simulink model "mpc_final"  (R2024a)
settings: Solver=ode4  StartTime=0  StopTime=5  FixedStep=0.25e-6  RelTol=1e-3
values from neighbouring files (symbols this model uses):
  B = 0    [PMSM_parameters.m]
  J = 0.006    [PMSM_parameters.m]
  Ls = 0.4    [PMSM_parameters.m]
  p = 4    [PMSM_parameters.m]
  Rs = 0.02    [PMSM_parameters.m]
  Sm = 0.2205    [PMSM_parameters.m]
libraries: slpidlib x4, embmathops x2, spsTHDLib x1
settings Model: NumberOfSteps=10  Creator=rohit  LastModifiedBy=rohit

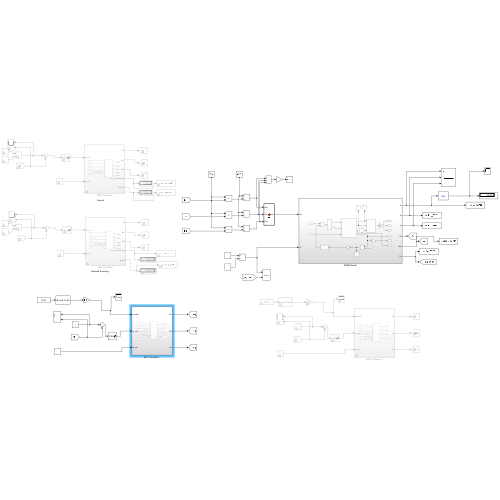
[thumbnail: Simulink's stored preview of the top-level diagram]
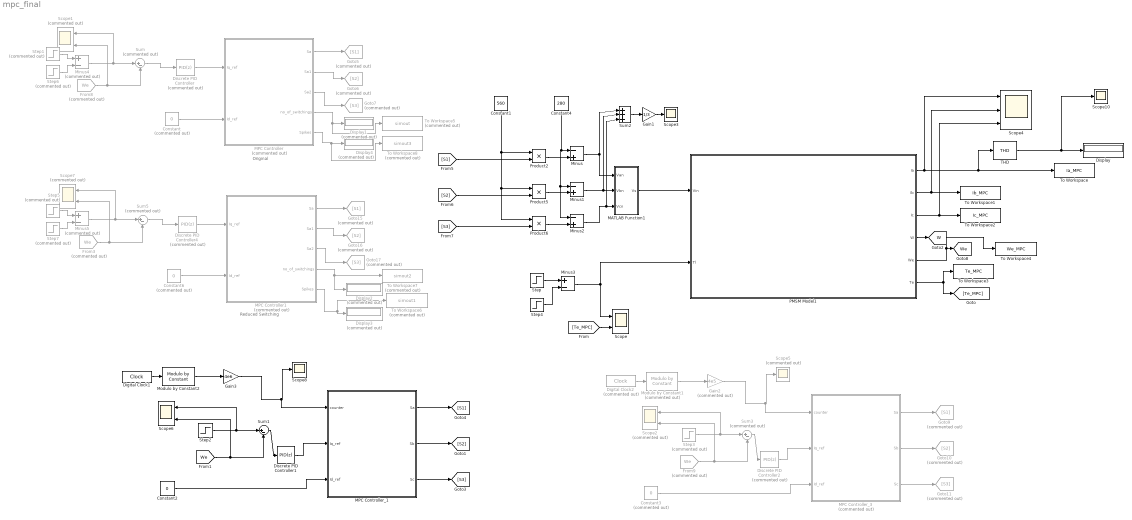
== system mpc_final ==
  note: Original
  note: Reduced Switching
  Constant : Constant  Commented=on  Value=0
  Constant1 : Constant  Value=560
  Constant2 : Constant  Value=0
  Constant3 : Constant  Commented=on  Value=0
  Constant4 : Constant  Value=280
  Constant6 : Constant  Commented=on  Value=0
  Digital Clock1 : DigitalClock  SampleTime=2.5e-6
  Digital Clock2 : DigitalClock  Commented=on  SampleTime=2.5e-6
  Discrete PID Controller : slpidlib/PID Controller  Commented=on  Controller=PID  Form=Parallel  TimeDomain=Discrete-time  UseExternalTs=off  SampleTime=-1  IntegratorMethod=Forward Euler  FilterMethod=Forward Euler  ControllerParametersSource=internal  P=10  I=1  UseKiTs=off  D=1  UseExternalDerivativeSource=off  N=100  UseFilter=off  TunerSelectOption=Transfer Function Based (PID Tuner App)  InitialConditionSource=internal  InitialConditionForIntegrator=0  InitialConditionForFilter=0  DifferentiatorICPrevScaledInput=0  ExternalReset=none  TrackingMode=off  Kt=1  LimitOutput=on  SatLimitsSource=internal  UpperSaturationLimit=90  LowerSaturationLimit=-90  LinearizeAsGain=on  AntiWindupMode=clamping  Kb=1  LimitIntegrator=off  UpperIntegratorSaturationLimit=inf  LowerIntegratorSaturationLimit=-inf  POutMin=[]  POutMax=[]  IOutMin=[]  IOutMax=[]  DOutMin=[]  DOutMax=[]  NOutMin=[]  NOutMax=[]  SumOutMin=[]  SumOutMax=[]  SaturationOutMin=[]  SaturationOutMax=[]  PParamMin=[]  PParamMax=[]  IParamMin=[]  IParamMax=[]  DParamMin=[]  DParamMax=[]  NParamMin=[]  NParamMax=[]  KbParamMin=[]  KbParamMax=[]  KtParamMin=[]  KtParamMax=[]  KbOutMin=[]  KbOutMax=[]  KtOutMin=[]  KtOutMax=[]  IntegratorOutMin=[]  IntegratorOutMax=[]  FilterOutMin=[]  FilterOutMax=[]  SumI1OutMin=[]  SumI1OutMax=[]  SumI2OutMin=[]  SumI2OutMax=[]  SumI3OutMin=[]  SumI3OutMax=[]  SumI4OutMin=[]  SumI4OutMax=[]  SumDOutMin=[]  SumDOutMax=[]  DifferentiatorOutMin=[]  DifferentiatorOutMax=[]  FilterDiffOutCoefMin=[]  FilterDiffOutCoefMax=[]  ReciprocalOutMin=[]  ReciprocalOutMax=[]  SumDenOutMin=[]  SumDenOutMax=[]  SumNumOutMin=[]  SumNumOutMax=[]  DivideOutMin=[]  DivideOutMax=[]  UdiffTsProdOutMin=[]  UdiffTsProdOutMax=[]  NTsProdOutMin=[]  NTsProdOutMax=[]  UintegralTsProdOutMin=[]  UintegralTsProdOutMax=[]  UngainTsProdOutMin=[]  UngainTsProdOutMax=[]  ClampingZeroOutDataTypeStr=Inherit: Inherit via back propagation  ClampingZeroOutMin=[]  ClampingZeroOutMax=[]  FilterDenConstantOutDataTypeStr=Inherit: Inherit via back propagation  FilterDenConstantOutMin=[]  FilterDenConstantOutMax=[]  PCopyOutDataTypeStr=Inherit: Inherit via back propagation  PCopyOutMin=[]  PCopyOutMax=[]  NCopyOutDataTypeStr=Inherit: Inherit via back propagation  NCopyOutMin=[]  NCopyOutMax=[]  IntegratorContinuousStateAttributes=''  IntegratorStateMustResolveToSignalObject=off  IntegratorRTWStateStorageClass=Auto  FilterContinuousStateAttributes=''  FilterStateMustResolveToSignalObject=off  FilterRTWStateStorageClass=Auto  ParallelPVariant=InternalParameters  IdealPVariant=Disabled  IVariant=InternalParameters  DVariant=InternalParameters  IntegratorVariant=Discrete  SatVariant=Enabled  AWVariant=DiscClampingParallel  PCopyVariant=Disabled  TRVariant=Disabled  FdbkBlocksVariant=Forward  IdealPFdbkVariant=Disabled  SatFdbkVariant=Disabled  DerivativeFilterVariant=Differentiator  NVariant=Passthrough  NCopyVariant=Disabled_SignalSpec  FilterICVariant=InternalICsDifferentiator  IntegratorICVariant=InternalICs  ExternalResetVariant=Disabled  TRSumVariant=Passthrough  SumFdbkVariant=Disabled  SumVariant=Sum_PID  TsampFilterVariant=InternalTs  TsampNgainVariant=Passthrough  TsampIntegralVariant=Disabled_SignalSpec  ExternalSaturationOutDataTypeStr=Inherit: Same as second input  DerivativeSourceVariant=ErrorSignal
  Discrete PID Controller1 : slpidlib/PID Controller  Controller=PID  Form=Parallel  TimeDomain=Discrete-time  UseExternalTs=off  SampleTime=-1  IntegratorMethod=Forward Euler  FilterMethod=Forward Euler  ControllerParametersSource=internal  P=10  I=1  UseKiTs=off  D=1  UseExternalDerivativeSource=off  N=100  UseFilter=off  TunerSelectOption=Transfer Function Based (PID Tuner App)  InitialConditionSource=internal  InitialConditionForIntegrator=0  InitialConditionForFilter=0  DifferentiatorICPrevScaledInput=0  ExternalReset=none  TrackingMode=off  Kt=1  LimitOutput=on  SatLimitsSource=internal  UpperSaturationLimit=90  LowerSaturationLimit=-90  LinearizeAsGain=on  AntiWindupMode=clamping  Kb=1  LimitIntegrator=off  UpperIntegratorSaturationLimit=inf  LowerIntegratorSaturationLimit=-inf  POutMin=[]  POutMax=[]  IOutMin=[]  IOutMax=[]  DOutMin=[]  DOutMax=[]  NOutMin=[]  NOutMax=[]  SumOutMin=[]  SumOutMax=[]  SaturationOutMin=[]  SaturationOutMax=[]  PParamMin=[]  PParamMax=[]  IParamMin=[]  IParamMax=[]  DParamMin=[]  DParamMax=[]  NParamMin=[]  NParamMax=[]  KbParamMin=[]  KbParamMax=[]  KtParamMin=[]  KtParamMax=[]  KbOutMin=[]  KbOutMax=[]  KtOutMin=[]  KtOutMax=[]  IntegratorOutMin=[]  IntegratorOutMax=[]  FilterOutMin=[]  FilterOutMax=[]  SumI1OutMin=[]  SumI1OutMax=[]  SumI2OutMin=[]  SumI2OutMax=[]  SumI3OutMin=[]  SumI3OutMax=[]  SumI4OutMin=[]  SumI4OutMax=[]  SumDOutMin=[]  SumDOutMax=[]  DifferentiatorOutMin=[]  DifferentiatorOutMax=[]  FilterDiffOutCoefMin=[]  FilterDiffOutCoefMax=[]  ReciprocalOutMin=[]  ReciprocalOutMax=[]  SumDenOutMin=[]  SumDenOutMax=[]  SumNumOutMin=[]  SumNumOutMax=[]  DivideOutMin=[]  DivideOutMax=[]  UdiffTsProdOutMin=[]  UdiffTsProdOutMax=[]  NTsProdOutMin=[]  NTsProdOutMax=[]  UintegralTsProdOutMin=[]  UintegralTsProdOutMax=[]  UngainTsProdOutMin=[]  UngainTsProdOutMax=[]  ClampingZeroOutDataTypeStr=Inherit: Inherit via back propagation  ClampingZeroOutMin=[]  ClampingZeroOutMax=[]  FilterDenConstantOutDataTypeStr=Inherit: Inherit via back propagation  FilterDenConstantOutMin=[]  FilterDenConstantOutMax=[]  PCopyOutDataTypeStr=Inherit: Inherit via back propagation  PCopyOutMin=[]  PCopyOutMax=[]  NCopyOutDataTypeStr=Inherit: Inherit via back propagation  NCopyOutMin=[]  NCopyOutMax=[]  IntegratorContinuousStateAttributes=''  IntegratorStateMustResolveToSignalObject=off  IntegratorRTWStateStorageClass=Auto  FilterContinuousStateAttributes=''  FilterStateMustResolveToSignalObject=off  FilterRTWStateStorageClass=Auto  ParallelPVariant=InternalParameters  IdealPVariant=Disabled  IVariant=InternalParameters  DVariant=InternalParameters  IntegratorVariant=Discrete  SatVariant=Enabled  AWVariant=DiscClampingParallel  PCopyVariant=Disabled  TRVariant=Disabled  FdbkBlocksVariant=Forward  IdealPFdbkVariant=Disabled  SatFdbkVariant=Disabled  DerivativeFilterVariant=Differentiator  NVariant=Passthrough  NCopyVariant=Disabled_SignalSpec  FilterICVariant=InternalICsDifferentiator  IntegratorICVariant=InternalICs  ExternalResetVariant=Disabled  TRSumVariant=Passthrough  SumFdbkVariant=Disabled  SumVariant=Sum_PID  TsampFilterVariant=InternalTs  TsampNgainVariant=Passthrough  TsampIntegralVariant=Disabled_SignalSpec  ExternalSaturationOutDataTypeStr=Inherit: Same as second input  DerivativeSourceVariant=ErrorSignal
  Discrete PID Controller2 : slpidlib/PID Controller  Commented=on  Controller=PID  Form=Parallel  TimeDomain=Discrete-time  UseExternalTs=off  SampleTime=-1  IntegratorMethod=Forward Euler  FilterMethod=Forward Euler  ControllerParametersSource=internal  P=10  I=1  UseKiTs=off  D=1  UseExternalDerivativeSource=off  N=100  UseFilter=off  TunerSelectOption=Transfer Function Based (PID Tuner App)  InitialConditionSource=internal  InitialConditionForIntegrator=0  InitialConditionForFilter=0  DifferentiatorICPrevScaledInput=0  ExternalReset=none  TrackingMode=off  Kt=1  LimitOutput=on  SatLimitsSource=internal  UpperSaturationLimit=90  LowerSaturationLimit=-90  LinearizeAsGain=on  AntiWindupMode=clamping  Kb=1  LimitIntegrator=off  UpperIntegratorSaturationLimit=inf  LowerIntegratorSaturationLimit=-inf  POutMin=[]  POutMax=[]  IOutMin=[]  IOutMax=[]  DOutMin=[]  DOutMax=[]  NOutMin=[]  NOutMax=[]  SumOutMin=[]  SumOutMax=[]  SaturationOutMin=[]  SaturationOutMax=[]  PParamMin=[]  PParamMax=[]  IParamMin=[]  IParamMax=[]  DParamMin=[]  DParamMax=[]  NParamMin=[]  NParamMax=[]  KbParamMin=[]  KbParamMax=[]  KtParamMin=[]  KtParamMax=[]  KbOutMin=[]  KbOutMax=[]  KtOutMin=[]  KtOutMax=[]  IntegratorOutMin=[]  IntegratorOutMax=[]  FilterOutMin=[]  FilterOutMax=[]  SumI1OutMin=[]  SumI1OutMax=[]  SumI2OutMin=[]  SumI2OutMax=[]  SumI3OutMin=[]  SumI3OutMax=[]  SumI4OutMin=[]  SumI4OutMax=[]  SumDOutMin=[]  SumDOutMax=[]  DifferentiatorOutMin=[]  DifferentiatorOutMax=[]  FilterDiffOutCoefMin=[]  FilterDiffOutCoefMax=[]  ReciprocalOutMin=[]  ReciprocalOutMax=[]  SumDenOutMin=[]  SumDenOutMax=[]  SumNumOutMin=[]  SumNumOutMax=[]  DivideOutMin=[]  DivideOutMax=[]  UdiffTsProdOutMin=[]  UdiffTsProdOutMax=[]  NTsProdOutMin=[]  NTsProdOutMax=[]  UintegralTsProdOutMin=[]  UintegralTsProdOutMax=[]  UngainTsProdOutMin=[]  UngainTsProdOutMax=[]  ClampingZeroOutDataTypeStr=Inherit: Inherit via back propagation  ClampingZeroOutMin=[]  ClampingZeroOutMax=[]  FilterDenConstantOutDataTypeStr=Inherit: Inherit via back propagation  FilterDenConstantOutMin=[]  FilterDenConstantOutMax=[]  PCopyOutDataTypeStr=Inherit: Inherit via back propagation  PCopyOutMin=[]  PCopyOutMax=[]  NCopyOutDataTypeStr=Inherit: Inherit via back propagation  NCopyOutMin=[]  NCopyOutMax=[]  IntegratorContinuousStateAttributes=''  IntegratorStateMustResolveToSignalObject=off  IntegratorRTWStateStorageClass=Auto  FilterContinuousStateAttributes=''  FilterStateMustResolveToSignalObject=off  FilterRTWStateStorageClass=Auto  ParallelPVariant=InternalParameters  IdealPVariant=Disabled  IVariant=InternalParameters  DVariant=InternalParameters  IntegratorVariant=Discrete  SatVariant=Enabled  AWVariant=DiscClampingParallel  PCopyVariant=Disabled  TRVariant=Disabled  FdbkBlocksVariant=Forward  IdealPFdbkVariant=Disabled  SatFdbkVariant=Disabled  DerivativeFilterVariant=Differentiator  NVariant=Passthrough  NCopyVariant=Disabled_SignalSpec  FilterICVariant=InternalICsDifferentiator  IntegratorICVariant=InternalICs  ExternalResetVariant=Disabled  TRSumVariant=Passthrough  SumFdbkVariant=Disabled  SumVariant=Sum_PID  TsampFilterVariant=InternalTs  TsampNgainVariant=Passthrough  TsampIntegralVariant=Disabled_SignalSpec  ExternalSaturationOutDataTypeStr=Inherit: Same as second input  DerivativeSourceVariant=ErrorSignal
  Discrete PID Controller4 : slpidlib/PID Controller  Commented=on  Controller=PID  Form=Parallel  TimeDomain=Discrete-time  UseExternalTs=off  SampleTime=-1  IntegratorMethod=Forward Euler  FilterMethod=Forward Euler  ControllerParametersSource=internal  P=10  I=1  UseKiTs=off  D=1  UseExternalDerivativeSource=off  N=100  UseFilter=off  TunerSelectOption=Transfer Function Based (PID Tuner App)  InitialConditionSource=internal  InitialConditionForIntegrator=0  InitialConditionForFilter=0  DifferentiatorICPrevScaledInput=0  ExternalReset=none  TrackingMode=off  Kt=1  LimitOutput=on  SatLimitsSource=internal  UpperSaturationLimit=90  LowerSaturationLimit=-90  LinearizeAsGain=on  AntiWindupMode=clamping  Kb=1  LimitIntegrator=off  UpperIntegratorSaturationLimit=inf  LowerIntegratorSaturationLimit=-inf  POutMin=[]  POutMax=[]  IOutMin=[]  IOutMax=[]  DOutMin=[]  DOutMax=[]  NOutMin=[]  NOutMax=[]  SumOutMin=[]  SumOutMax=[]  SaturationOutMin=[]  SaturationOutMax=[]  PParamMin=[]  PParamMax=[]  IParamMin=[]  IParamMax=[]  DParamMin=[]  DParamMax=[]  NParamMin=[]  NParamMax=[]  KbParamMin=[]  KbParamMax=[]  KtParamMin=[]  KtParamMax=[]  KbOutMin=[]  KbOutMax=[]  KtOutMin=[]  KtOutMax=[]  IntegratorOutMin=[]  IntegratorOutMax=[]  FilterOutMin=[]  FilterOutMax=[]  SumI1OutMin=[]  SumI1OutMax=[]  SumI2OutMin=[]  SumI2OutMax=[]  SumI3OutMin=[]  SumI3OutMax=[]  SumI4OutMin=[]  SumI4OutMax=[]  SumDOutMin=[]  SumDOutMax=[]  DifferentiatorOutMin=[]  DifferentiatorOutMax=[]  FilterDiffOutCoefMin=[]  FilterDiffOutCoefMax=[]  ReciprocalOutMin=[]  ReciprocalOutMax=[]  SumDenOutMin=[]  SumDenOutMax=[]  SumNumOutMin=[]  SumNumOutMax=[]  DivideOutMin=[]  DivideOutMax=[]  UdiffTsProdOutMin=[]  UdiffTsProdOutMax=[]  NTsProdOutMin=[]  NTsProdOutMax=[]  UintegralTsProdOutMin=[]  UintegralTsProdOutMax=[]  UngainTsProdOutMin=[]  UngainTsProdOutMax=[]  ClampingZeroOutDataTypeStr=Inherit: Inherit via back propagation  ClampingZeroOutMin=[]  ClampingZeroOutMax=[]  FilterDenConstantOutDataTypeStr=Inherit: Inherit via back propagation  FilterDenConstantOutMin=[]  FilterDenConstantOutMax=[]  PCopyOutDataTypeStr=Inherit: Inherit via back propagation  PCopyOutMin=[]  PCopyOutMax=[]  NCopyOutDataTypeStr=Inherit: Inherit via back propagation  NCopyOutMin=[]  NCopyOutMax=[]  IntegratorContinuousStateAttributes=''  IntegratorStateMustResolveToSignalObject=off  IntegratorRTWStateStorageClass=Auto  FilterContinuousStateAttributes=''  FilterStateMustResolveToSignalObject=off  FilterRTWStateStorageClass=Auto  ParallelPVariant=InternalParameters  IdealPVariant=Disabled  IVariant=InternalParameters  DVariant=InternalParameters  IntegratorVariant=Discrete  SatVariant=Enabled  AWVariant=DiscClampingParallel  PCopyVariant=Disabled  TRVariant=Disabled  FdbkBlocksVariant=Forward  IdealPFdbkVariant=Disabled  SatFdbkVariant=Disabled  DerivativeFilterVariant=Differentiator  NVariant=Passthrough  NCopyVariant=Disabled_SignalSpec  FilterICVariant=InternalICsDifferentiator  IntegratorICVariant=InternalICs  ExternalResetVariant=Disabled  TRSumVariant=Passthrough  SumFdbkVariant=Disabled  SumVariant=Sum_PID  TsampFilterVariant=InternalTs  TsampNgainVariant=Passthrough  TsampIntegralVariant=Disabled_SignalSpec  ExternalSaturationOutDataTypeStr=Inherit: Same as second input  DerivativeSourceVariant=ErrorSignal
  Display : Display
  Display{1..4} (4 alike) : Display  Commented=on
  From3 : From  Commented=on  GotoTag=We  TagVisibility=global
  From8 : From  Commented=on  GotoTag=We  TagVisibility=global
  From9 : From  Commented=on  GotoTag=We  TagVisibility=global
  Gain1 : Gain  Gain=1/3
  Gain2 : Gain  Commented=on  Gain=4e5
  Gain3 : Gain  Gain=4e6
  Goto10 : Goto  Commented=on  GotoTag=S2
  Goto11 : Goto  Commented=on  GotoTag=S3
  Goto15 : Goto  Commented=on  GotoTag=S1
  Goto16 : Goto  Commented=on  GotoTag=S2
  Goto17 : Goto  Commented=on  GotoTag=S3
  Goto5 : Goto  Commented=on  GotoTag=S1
  Goto6 : Goto  Commented=on  GotoTag=S2
  Goto7 : Goto  Commented=on  GotoTag=S3
  Goto9 : Goto  Commented=on  GotoTag=S1
  MATLAB Function1 : MATLAB Function  TreatAsAtomicUnit=on
  MPC Controller : Subsystem  Commented=on
  MPC Controller1 : Subsystem  Commented=on
  MPC Controller_1 : Subsystem
  MPC Controller_3 : Subsystem  Commented=on
  Minus : Sum  Inputs=-+
  Minus1 : Sum  Inputs=-+
  Minus2 : Sum  Inputs=-+
  Minus3 : Sum  Inputs=+-
  Minus4 : Sum  Commented=on  Inputs=+-
  Minus5 : Sum  Commented=on  Inputs=+-
  Modulo by Constant1 : embmathops/Modulo by Constant  Commented=on  Denominator=10e-6  SimulateUsing=Code generation
      settings: LibrarySourceBlock=embeddedMathLib/Modulo by Constant
  Modulo by Constant2 : embmathops/Modulo by Constant  Denominator=1e-6  SimulateUsing=Code generation
      settings: LibrarySourceBlock=embeddedMathLib/Modulo by Constant
  PMSM Model1 : Subsystem
  Product2 : Product
  Product5 : Product
  Product6 : Product
  Scope : Scope  NumInputPorts=2
  Scope1 : Scope  Commented=on  NumInputPorts=2
  Scope10 : Scope
  Scope2 : Scope  Commented=on  NumInputPorts=2
  Scope3 : Scope
  Scope4 : Scope  NumInputPorts=3
  Scope5 : Scope  Commented=on
  Scope6 : Scope  NumInputPorts=2
  Scope7 : Scope  Commented=on  NumInputPorts=2
  Scope8 : Scope
  Step : Step  Time=2.5  After=200  SampleTime=0
  Step1 : Step  Commented=on  Time=1.5  Before=100  After=200  SampleTime=0
  Step2 : Step  Time=2  Before=200  After=400  SampleTime=0
  Step3 : Step  Commented=on  Time=2  Before=200  After=400  SampleTime=0
  Step4 : Step  Time=3  After=0  SampleTime=0
  Step5 : Step  Commented=on  Time=1.5  Before=100  After=200  SampleTime=0
  Step6 : Step  Commented=on  Time=3.5  After=100  SampleTime=0
  Step7 : Step  Commented=on  Time=3.5  After=100  SampleTime=0
  Sum : Sum  Commented=on  Inputs=|+-
  Sum1 : Sum  Inputs=|+-
  Sum2 : Sum  Inputs=|+++
  Sum3 : Sum  Commented=on  Inputs=|+-
  Sum5 : Sum  Commented=on  Inputs=|+-
  THD : spsTHDLib/THD  Freq=100/12  Ts=0
  To Workspace : ToWorkspace  VariableName=Ia_MPC  SaveFormat=Timeseries  SampleTime=-1
  To Workspace1 : ToWorkspace  VariableName=Ib_MPC  SaveFormat=Timeseries  SampleTime=-1
  To Workspace2 : ToWorkspace  VariableName=Ic_MPC  SaveFormat=Timeseries  SampleTime=-1
  To Workspace3 : ToWorkspace  VariableName=Te_MPC  SaveFormat=Timeseries  SampleTime=-1
  To Workspace4 : ToWorkspace  VariableName=We_MPC  SaveFormat=Timeseries  SampleTime=-1
  To Workspace5 : ToWorkspace  Commented=on  VariableName=simout  SaveFormat=Timeseries  SampleTime=-1
  To Workspace6 : ToWorkspace  Commented=on  VariableName=simout1  SaveFormat=Timeseries  SampleTime=-1
  To Workspace7 : ToWorkspace  Commented=on  VariableName=simout2  SaveFormat=Timeseries  SampleTime=-1
  To Workspace8 : ToWorkspace  Commented=on  VariableName=simout3  SaveFormat=Timeseries  SampleTime=-1
  tag scope: W=global, We=global
  wires:
  Minus2/1 -> Sum2/3, MATLAB Function1/3(Vcn)
  [S3] -> Product6/2
  Constant4/1 -> Minus2/1, Minus1/1, Minus/1
  Product2/1 -> Minus/2
  Minus/1 -> Sum2/1, MATLAB Function1/1(Van)
  [S1] -> Product2/2
  [Te_MPC] -> Scope/2
  PMSM Model1/1(Ia) -> THD/1, To Workspace/1, Scope4/1
  Product6/1 -> Minus2/2
  Gain1/1 -> Scope3/1
  Product5/1 -> Minus1/2
  Sum/1 -> Discrete PID Controller/1
  Minus3/1 -> PMSM Model1/2(Tl), Scope/1
  Discrete PID Controller/1 -> MPC Controller/1(Iq_ref)
  PMSM Model1/5(We) -> To Workspace4/1, [We]
  PMSM Model1/4(W) -> [W]
  [S2] -> Product5/2
  Constant1/1 -> Product2/1, Product5/1, Product6/1
  PMSM Model1/3(Ic) -> Scope4/3, To Workspace2/1
  PMSM Model1/2(Ib) -> Scope4/2, To Workspace1/1
  MATLAB Function1/1(Vs) -> PMSM Model1/1(Vin)
  Sum2/1 -> Gain1/1
  PMSM Model1/6(Te) -> To Workspace3/1, [Te_MPC]
  Constant/1 -> MPC Controller/2(Id_ref)
  Minus1/1 -> Sum2/2, MATLAB Function1/2(Vbn)
  From8/1 -> Sum/2, Scope1/2
  Minus4/1 -> Scope1/1, Sum/1
  MPC Controller/1(Sa) -> Goto5/1
  MPC Controller/2(Sa1) -> Goto6/1
  MPC Controller/3(Sa2) -> Goto7/1
  MPC Controller_3/3(Sc) -> Goto11/1
  From9/1 -> Scope2/2, Sum3/2
  MPC Controller_3/2(Sb) -> Goto10/1
  Digital Clock2/1 -> Modulo by Constant1/1
  Sum3/1 -> Discrete PID Controller2/1
  Gain2/1 -> MPC Controller_3/1(counter), Scope5/1
  Step3/1 -> Scope2/1, Sum3/1
  Constant3/1 -> MPC Controller_3/3(Id_ref)
  Modulo by Constant1/1 -> Gain2/1
  Discrete PID Controller2/1 -> MPC Controller_3/2(Iq_ref)
  MPC Controller_3/1(Sa) -> Goto9/1
  MPC Controller/4(no_of_switchings) -> To Workspace5/1, Display1/1
  MPC Controller1/4(no_of_switchings) -> Display2/1, To Workspace7/1
  Discrete PID Controller4/1 -> MPC Controller1/1(Iq_ref)
  Minus5/1 -> Scope7/1, Sum5/1
  MPC Controller1/3(Sa2) -> Goto17/1
  Constant6/1 -> MPC Controller1/2(Id_ref)
  MPC Controller1/2(Sa1) -> Goto16/1
  MPC Controller1/1(Sa) -> Goto15/1
  Sum5/1 -> Discrete PID Controller4/1
  From3/1 -> Sum5/2, Scope7/2
  THD/1 -> Scope10/1, Display/1
  Sum1/1 -> Discrete PID Controller1/1
  Constant2/1 -> MPC Controller_1/3(Id_ref)
  Modulo by Constant2/1 -> Gain3/1
  MPC Controller_1/3(Sc) -> [S3]
  MPC Controller_1/1(Sa) -> [S1]
  Discrete PID Controller1/1 -> MPC Controller_1/2(Iq_ref)
  Step2/1 -> Scope6/1, Sum1/1
  MPC Controller_1/2(Sb) -> [S2]
  [We] -> Scope6/2, Sum1/2
  Digital Clock1/1 -> Modulo by Constant2/1
  Gain3/1 -> MPC Controller_1/1(counter), Scope8/1
  MPC Controller1/5(Spikes) -> Display3/1, To Workspace6/1
  MPC Controller/5(Spikes) -> To Workspace8/1, Display4/1
  Step/1 -> Minus3/1
  Step4/1 -> Minus3/2
  Step1/1 -> Minus4/1
  Step6/1 -> Minus4/2
  Step7/1 -> Minus5/2
  Step5/1 -> Minus5/1

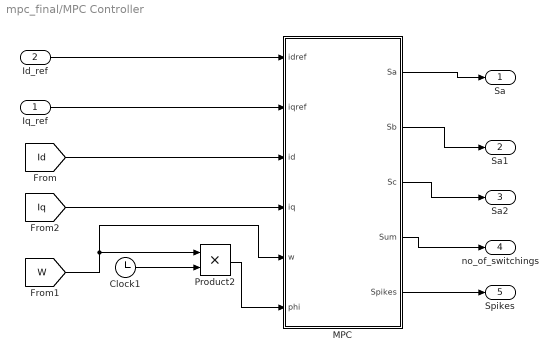
== system mpc_final/MPC Controller ==
  Iq_ref : Inport
  Id_ref : Inport  Port=2
  Clock1 : Clock
  MPC : MATLAB Function  TreatAsAtomicUnit=on
  Product2 : Product
  Sa : Outport
  Sa1 : Outport  Port=2
  Sa2 : Outport  Port=3
  no_of_switchings : Outport  Port=4
  Spikes : Outport  Port=5
  wires:
  Clock1/1 -> Product2/2
  [Iq] -> MPC/4(iq)
  [Id] -> MPC/3(id)
  Iq_ref/1 -> MPC/2(iqref)
  Id_ref/1 -> MPC/1(idref)
  Product2/1 -> MPC/6(phi)
  [W] -> Product2/1, MPC/5(w)
  MPC/1(Sa) -> Sa/1
  MPC/2(Sb) -> Sa1/1
  MPC/3(Sc) -> Sa2/1
  MPC/4(Sum) -> no_of_switchings/1
  MPC/5(Spikes) -> Spikes/1

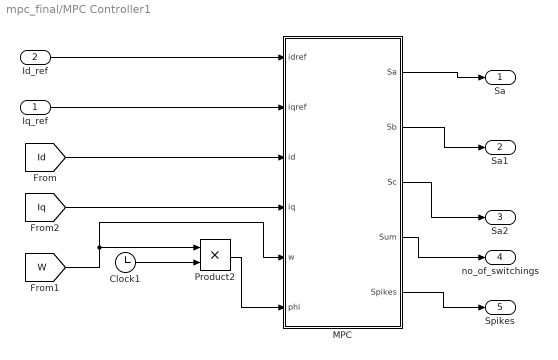
== system mpc_final/MPC Controller1 ==
  Iq_ref : Inport
  Id_ref : Inport  Port=2
  Clock1 : Clock
  MPC : MATLAB Function  TreatAsAtomicUnit=on
  Product2 : Product
  Sa : Outport
  Sa1 : Outport  Port=2
  Sa2 : Outport  Port=3
  no_of_switchings : Outport  Port=4
  Spikes : Outport  Port=5
  wires:
  Clock1/1 -> Product2/2
  [Iq] -> MPC/4(iq)
  [Id] -> MPC/3(id)
  Iq_ref/1 -> MPC/2(iqref)
  Id_ref/1 -> MPC/1(idref)
  Product2/1 -> MPC/6(phi)
  [W] -> Product2/1, MPC/5(w)
  MPC/1(Sa) -> Sa/1
  MPC/2(Sb) -> Sa1/1
  MPC/3(Sc) -> Sa2/1
  MPC/4(Sum) -> no_of_switchings/1
  MPC/5(Spikes) -> Spikes/1

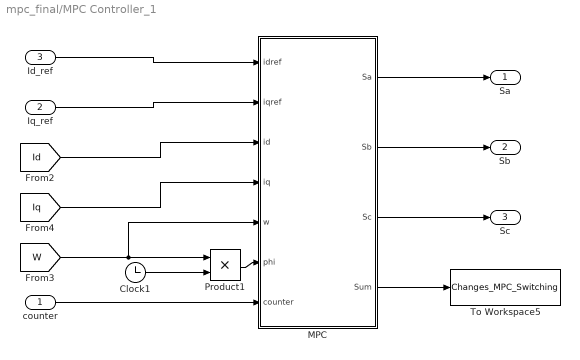
== system mpc_final/MPC Controller_1 ==
  counter : Inport
  Iq_ref : Inport  Port=2
  Id_ref : Inport  Port=3
  Clock1 : Clock
  MPC : MATLAB Function  TreatAsAtomicUnit=on
  Product1 : Product
  To Workspace5 : ToWorkspace  VariableName=Changes_MPC_Switching  SaveFormat=Timeseries  SampleTime=-1
  Sa : Outport
  Sb : Outport  Port=2
  Sc : Outport  Port=3
  wires:
  MPC/2(Sb) -> Sb/1
  Id_ref/1 -> MPC/1(idref)
  MPC/4(Sum) -> To Workspace5/1
  Iq_ref/1 -> MPC/2(iqref)
  Clock1/1 -> Product1/2
  Product1/1 -> MPC/6(phi)
  [Iq] -> MPC/4(iq)
  [Id] -> MPC/3(id)
  MPC/3(Sc) -> Sc/1
  MPC/1(Sa) -> Sa/1
  [W] -> MPC/5(w), Product1/1
  counter/1 -> MPC/7(counter)

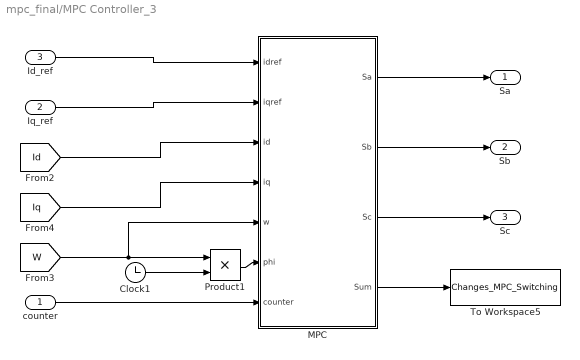
== system mpc_final/MPC Controller_3 ==
  counter : Inport
  Iq_ref : Inport  Port=2
  Id_ref : Inport  Port=3
  Clock1 : Clock
  MPC : MATLAB Function  TreatAsAtomicUnit=on
  Product1 : Product
  To Workspace5 : ToWorkspace  VariableName=Changes_MPC_Switching  SaveFormat=Timeseries  SampleTime=-1
  Sa : Outport
  Sb : Outport  Port=2
  Sc : Outport  Port=3
  wires:
  MPC/2(Sb) -> Sb/1
  Id_ref/1 -> MPC/1(idref)
  MPC/4(Sum) -> To Workspace5/1
  Iq_ref/1 -> MPC/2(iqref)
  Clock1/1 -> Product1/2
  Product1/1 -> MPC/6(phi)
  [Iq] -> MPC/4(iq)
  [Id] -> MPC/3(id)
  MPC/3(Sc) -> Sc/1
  MPC/1(Sa) -> Sa/1
  [W] -> MPC/5(w), Product1/1
  counter/1 -> MPC/7(counter)

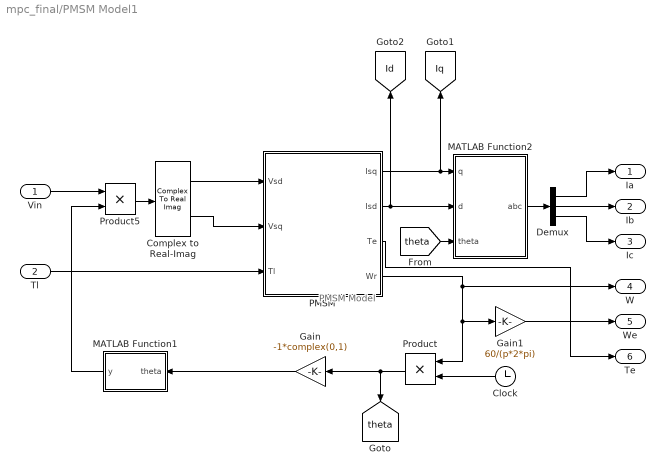
== system mpc_final/PMSM Model1 ==
  note: PMSM Model
  Vin : Inport
  Tl : Inport  Port=2
  Clock : Clock
  Complex to Real-Imag : ComplexToRealImag
  Demux : Demux  Outputs=3
  Gain : Gain  Gain=-1*complex(0,1)
  Gain1 : Gain  Gain=60/(p*2*pi)
  MATLAB Function1 : MATLAB Function  TreatAsAtomicUnit=on
  MATLAB Function2 : MATLAB Function  TreatAsAtomicUnit=on
  PMSM : Subsystem
  Product : Product
  Product5 : Product
  Ia : Outport
  Ib : Outport  Port=2
  Ic : Outport  Port=3
  W : Outport  Port=4
  We : Outport  Port=5
  Te : Outport  Port=6
  tag scope: Id=global, Iq=global, theta=global
  wires:
  Tl/1 -> PMSM/3(Tl)
  PMSM/4(Wr) -> W/1, Gain1/1, Product/1
  Product/1 -> Gain/1, [theta]
  Demux/3 -> Ic/1
  Clock/1 -> Product/2
  PMSM/1(Isq) -> [Iq], MATLAB Function2/1(q)
  MATLAB Function1/1(y) -> Product5/2
  Complex to Real-Imag/1 -> PMSM/1(Vsd)
  PMSM/3(Te) -> Te/1
  PMSM/2(Isd) -> MATLAB Function2/2(d), [Id]
  Complex to Real-Imag/2 -> PMSM/2(Vsq)
  Product5/1 -> Complex to Real-Imag/1
  Gain/1 -> MATLAB Function1/1(theta)
  Demux/1 -> Ia/1
  MATLAB Function2/1(abc) -> Demux/1
  Vin/1 -> Product5/1
  Gain1/1 -> We/1
  Demux/2 -> Ib/1
  [theta] -> MATLAB Function2/3(theta)

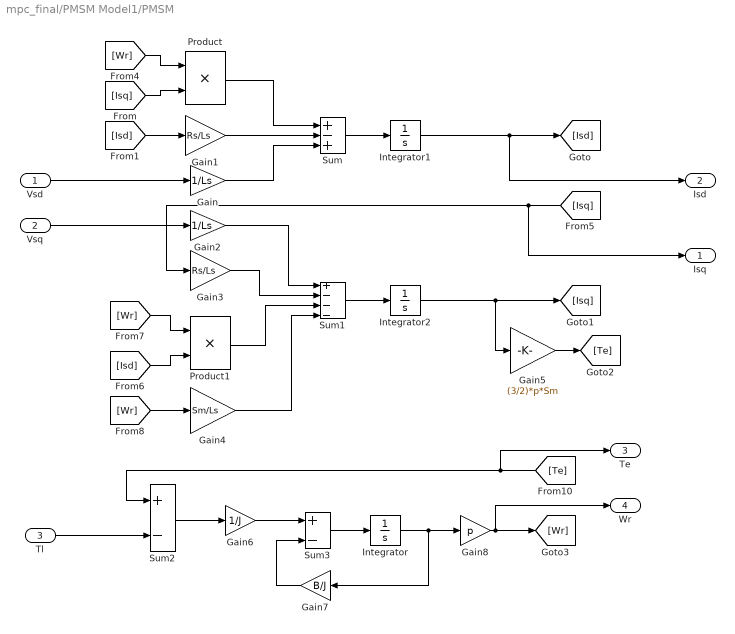
== system mpc_final/PMSM Model1/PMSM ==
  Vsd : Inport
  Vsq : Inport  Port=2
  Tl : Inport  Port=3
  Gain : Gain  Gain=1/Ls
  Gain1 : Gain  Gain=Rs/Ls
  Gain2 : Gain  Gain=1/Ls
  Gain3 : Gain  Gain=Rs/Ls
  Gain4 : Gain  Gain=Sm/Ls
  Gain5 : Gain  Gain=(3/2)*p*Sm
  Gain6 : Gain  Gain=1/J
  Gain7 : Gain  Gain=B/J
  Gain8 : Gain  Gain=p
  Integrator : Integrator
  Integrator1 : Integrator
  Integrator2 : Integrator
  Product : Product
  Product1 : Product
  Sum : Sum  Inputs=+-+
  Sum1 : Sum  Inputs=+---
  Sum2 : Sum  Inputs=+-
  Sum3 : Sum  Inputs=+-
  Isq : Outport
  Isd : Outport  Port=2
  Te : Outport  Port=3
  Wr : Outport  Port=4
  wires:
  Gain5/1 -> [Te]
  [Wr] -> Gain4/1
  [Isq] -> Isq/1, Gain3/1
  [Te] -> Te/1, Sum2/1
  Integrator2/1 -> Gain5/1, [Isq]
  Gain6/1 -> Sum3/1
  Sum1/1 -> Integrator2/1
  Gain/1 -> Sum/3
  Integrator/1 -> Gain8/1, Gain7/1
  Tl/1 -> Sum2/2
  Gain8/1 -> Wr/1, [Wr]
  Gain2/1 -> Sum1/1
  Sum3/1 -> Integrator/1
  Vsd/1 -> Gain/1
  Sum2/1 -> Gain6/1
  [Isd] -> Product1/2
  Gain7/1 -> Sum3/2
  Gain3/1 -> Sum1/2
  Gain4/1 -> Sum1/4
  [Wr] -> Product/1
  [Isq] -> Product/2
  Product1/1 -> Sum1/3
  [Wr] -> Product1/1
  Product/1 -> Sum/1
  Gain1/1 -> Sum/2
  [Isd] -> Gain1/1
  Sum/1 -> Integrator1/1
  Vsq/1 -> Gain2/1
  Integrator1/1 -> Isd/1, [Isd]

== matlab function mpc_final/PMSM Model1/MATLAB Function1 ==
  data: theta input; y output
function y = fcn(theta)

y = exp((theta));

== matlab function mpc_final/PMSM Model1/MATLAB Function2 ==
  data: q input; d input; abc output; theta input
function abc = dq_to_abc(q, d, theta)
    % Inputs:
    % d, q   : DQ components
    % theta  : Electrical angle in radians

    % Transformation matrix
    T = [cos(theta), -sin(theta), 1; 
         cos(theta - 2*pi/3), -sin(theta - 2*pi/3), 1; 
         cos(theta + 2*pi/3), -sin(theta + 2*pi/3), 1];

    % Calculate abc components
    abc = (2/3) * T * [d; q; 0];
end

== matlab function mpc_final/MPC Controller_3/MPC ==
  settings: updateMethod=DISCRETE
  data: idref input; Sa output; iqref input; id input; iq input; w input; Sb output; Sc output; phi input; Sum output; counter input
function [Sa, Sb, Sc, Sum] = mpc(idref, iqref, id, iq, w, phi,counter) 
    %% Initialisation 
    R = 0.02;
    Ls = 0.4;
    Vdc = 500;
    Lambda_f = 0.2205;
    Ts = 10e-6;
    imax = 80;
    p = 4;
    cost = 1e14; 
    % switching_weight = 1e3; % Weight factor for switching losses
    
    persistent state prev_state; 
    if isempty(state) 
        state = 1;
        prev_state = 1; % Store previous switching state
    end
    persistent sum ; 
    if isempty(sum)
        sum = 0;
    end
    
    S = [0 0 0; 1 0 0; 1 1 0; 0 1 0; 0 1 1; 0 0 1; 1 0 1; 1 1 1]; 

    if counter == 0
        prev_state = state ;
        for i = 1:8
            ud = Vdc * (2/3) * (S(i,1)*cos(phi) + S(i,2)*cos(phi-2*pi/3) + S(i,3)*cos(phi + 2*pi/3)); 
            uq = Vdc * (2/3) * (-S(i,1) * sin(phi) - S(i,2) * sin(phi- 2*pi/3) - S(i,3) * sin(phi + 2*pi/3));
            
            id1 = ((1 - (R*Ts)/Ls) * id) + ((Ts * ud) / Ls) + (w * Ts * iq); 
            iq1 = ((1 - (R*Ts)/Ls) * iq) + ((Ts * uq) / Ls) - ((w * Ts * id)) - (((w * Ts * Lambda_f) / Ls)); 
            
            f = 0; 
            if abs(id1) > imax || abs(iq1) > imax 
                f = 1e14; 
            end
            
            % Switching loss penalty
            switch_changes = (S(i,1)-S(prev_state,1))^2+(S(i,2)-S(prev_state,2))^2+(S(i,3)-S(prev_state,3))^2 ; % Count switch state changes\
            f_switching = 0;
            if switch_changes > 1
                f_switching = 1e5;
            end
            
            current_cost = (idref - id1)^2 + (iqref - iq1)^2 + f + f_switching;  
            
            if current_cost < cost 
                state = i;
                cost = current_cost;
            end
        end
        if((state == 1)||(state == 8))
            sum = sum + 6 ;
        else
            sum = sum + (S(state,1)-S(prev_state,1))^2+(S(state,2)-S(prev_state,2))^2+(S(state,3)-S(prev_state,3))^2;
        end
    end

    if(state == 8 || state == 1)
        if(counter == 0)
            Sa = S(prev_state,1);
            Sb = S(prev_state,2);
            Sc = S(prev_state,3);
        elseif(counter == 1)
            Sa = 1-S(prev_state,1);
            Sb = 1-S(prev_state,2);
            Sc = 1-S(prev_state,3);
        elseif(counter == 2)
            Sa = 1-S(prev_state,1);
            Sb = 1-S(prev_state,2);
            Sc = 1-S(prev_state,3);
        else
            Sa = S(prev_state,1);
            Sb = S(prev_state,2);
            Sc = S(prev_state,3);
        end
    else
        Sa = S(state,1);
        Sb = S(state,2);
        Sc = S(state,3);
    end

    Sum = sum;
end

== matlab function mpc_final/MPC Controller_1/MPC ==
  settings: updateMethod=DISCRETE
  data: idref input; Sa output; iqref input; id input; iq input; w input; Sb output; Sc output; phi input; Sum output; counter input
function [Sa, Sb, Sc, Sum] = mpc(idref, iqref, id, iq, w, phi,counter) 
    %% Initialisation 
    R = 0.02;
    Ls = 0.4;
    Vdc = 500;
    Lambda_f = 0.2205;
    Ts = 1e-6;
    imax = 80;
    p = 4;
    cost = 1e14; 
    % switching_weight = 1e3; % Weight factor for switching losses
    
    persistent state prev_state; 
    if isempty(state) 
        state = 1;
        prev_state = 1; % Store previous switching state
    end
    persistent sum ; 
    if isempty(sum)
        sum = 0;
    end
    
    S = [0 0 0; 1 0 0; 1 1 0; 0 1 0; 0 1 1; 0 0 1; 1 0 1; 1 1 1]; 

    if counter == 0
        prev_state = state ;
        for i = 1:8
            ud = Vdc * (2/3) * (S(i,1)*cos(phi) + S(i,2)*cos(phi-2*pi/3) + S(i,3)*cos(phi + 2*pi/3)); 
            uq = Vdc * (2/3) * (-S(i,1) * sin(phi) - S(i,2) * sin(phi- 2*pi/3) - S(i,3) * sin(phi + 2*pi/3));
            id1 = ((1 - (R*Ts)/Ls) * id) + ((Ts * ud) / Ls) + (w * Ts * iq); 
            iq1 = ((1 - (R*Ts)/Ls) * iq) + ((Ts * uq) / Ls) - ((w * Ts * id)) - (((w * Ts * Lambda_f) / Ls)); 
            f = 0; 
            if abs(id1) > imax || abs(iq1) > imax 
                f = 1e14; 
            end
            current_cost = (idref - id1)^2 + (iqref - iq1)^2 + f ;  
            if current_cost < cost 
                state = i;
                cost = current_cost;
            end
        end

        if((state == 1)||(state == 8))
            sum = sum + 6 ;
        else
            sum = sum + (S(state,1)-S(prev_state,1))^2+(S(state,2)-S(prev_state,2))^2+(S(state,3)-S(prev_state,3))^2;
        end
        
    end

    if(state == 8 || state == 1)
        if(counter == 0)
            Sa = S(prev_state,1);
            Sb = S(prev_state,2);
            Sc = S(prev_state,3);
        elseif(counter == 1)
            Sa = 1-S(prev_state,1);
            Sb = 1-S(prev_state,2);
            Sc = 1-S(prev_state,3);
        elseif(counter == 2)
            Sa = 1-S(prev_state,1);
            Sb = 1-S(prev_state,2);
            Sc = 1-S(prev_state,3);
        else
            Sa = S(prev_state,1);
            Sb = S(prev_state,2);
            Sc = S(prev_state,3);
        end
    else
        Sa = S(state,1);
        Sb = S(state,2);
        Sc = S(state,3);
    end

    Sum = sum;
end

== matlab function mpc_final/MPC Controller/MPC ==
  settings: updateMethod=DISCRETE
  data: idref input; Sa output; iqref input; id input; iq input; w input; Sb output; Sc output; phi input; Sum output; Spikes output
function [Sa, Sb, Sc,Sum,Spikes] = mpc(idref, iqref, id, iq, w,phi) 
    %% Initialisation 
    % R = 0.02;
    % Ls = 0.4;
    Vdc = 560;
    % Lambda_f = 0.2205;
    Ts = 1e-6;
    imax=300;
    % p=4;
    R = 87e-3 ;
    Ls = 0.8e-3;
    Lambda_f = 0.5; %Sm is phi_r or flux linkage
    p = 5; %pole pair

    cost=1e14; 
    persistent state prev_state x y; 

    if isempty(x)
        x = 0; 
    end
    if isempty(y)
        y=0;
    end
    if isempty(state)
        state = 1; 
        prev_state = 1;
    end

    S = [0 0 0 ; 1 0 0; 1 1 0; 0 1 0; 0 1 1; 0 0 1; 1 0 1 ; 1 1 1]; 
    prev_state = state ;
    for i=1:8
        ud = Vdc*(2/3)*(S(i,1)*cos(phi) + S(i,2)*cos(phi-2*pi/3) + S(i,3)*cos(phi + 2*pi/3)); 
        uq = Vdc*(2/3)* (-S(i,1) *sin(phi) - S(i,2)*sin(phi- 2*pi/3) - S(i,3)*sin(phi + 2*pi/3));
        id1 = ((1 -(R*Ts)/Ls)*id) + ((Ts*ud)/Ls) + (w*Ts*iq) ; 
        iq1 = ((1 - (R*Ts)/Ls)*iq) + ((Ts*uq)/Ls) - ((w*Ts*id)) - (((w*Ts*Lambda_f)/1)); 
        f = 0; 
        if abs(id1) > imax || abs(iq1) > imax 
            f = 1e14; 
        end
        current_cost=(idref-id1)^2 + (iqref-iq1)^2 +f; 
        if(current_cost<cost) 
            state=i;
            cost=current_cost;
        end
    end

    Sa = S(state,1);
    Sb = S(state,2); 
    Sc = S(state,3);

    Sap = S(prev_state,1);
    Sbp = S(prev_state,2); 
    Scp = S(prev_state,3);

    x = x + (Sa-Sap)^2 + (Sb-Sbp)^2 + (Sc-Scp)^2 ;

    if ((state == 1 || state == 8) && (prev_state~=state))
        y = y + 1;
    end

    Sum = x ;
    Spikes = y;
end

== matlab function mpc_final/MPC Controller1/MPC ==
  settings: updateMethod=DISCRETE
  data: idref input; Sa output; iqref input; id input; iq input; w input; Sb output; Sc output; phi input; Sum output; Spikes output
function [Sa, Sb, Sc,Sum,Spikes] = mpc(idref, iqref, id, iq, w,phi) 
    %% Initialisation 
    R = 0.02;
    Ls = 0.4;
    Vdc = 500;
    Lambda_f = 0.2205;
    Ts = 10e-6;
    imax=80;
    p=4;
    cost=1e14; 
    persistent state prev_state x y; 

    if isempty(x)
        x = 0; 
    end
    if isempty(y)
        y = 0;
    end
    if isempty(state)
        state = 1; 
        prev_state = 1;
    end

    S = [0 0 0 ; 1 0 0; 1 1 0; 0 1 0; 0 1 1; 0 0 1; 1 0 1 ; 1 1 1]; 
    prev_state = state ;
    Sap = S(prev_state,1);
    Sbp = S(prev_state,2); 
    Scp = S(prev_state,3);

    for i=1:8    
        ud = Vdc * (2/3) * (S(i,1)*cos(phi) + S(i,2)*cos(phi-2*pi/3) + S(i,3)*cos(phi + 2*pi/3)); 
        uq = Vdc * (2/3) * (-S(i,1) * sin(phi) - S(i,2) * sin(phi- 2*pi/3) - S(i,3) * sin(phi + 2*pi/3));
        id1 = ((1 - (R*Ts)/Ls) * id) + ((Ts * ud) / Ls) + (w * Ts * iq); 
        iq1 = ((1 - (R*Ts)/Ls) * iq) + ((Ts * uq) / Ls) - ((w * Ts * id)) - (((w * Ts * Lambda_f) / Ls));
        f = 0; 
        if abs(id1) > imax || abs(iq1) > imax 
            f = 1e14; 
        end
        
        % Switching loss penalty
        switch_changes = (Sap-S(i,1))^2 + (Sbp-S(i,2))^2 + (Scp-S(i,3))^2; % Count switch state changes\
        f_switching = 0;
        if switch_changes > 1
            f_switching = 1e5;
        end
        
        current_cost = (idref - id1)^2 + (iqref - iq1)^2 + f + f_switching;  
        if current_cost < cost 
            state = i;
            cost = current_cost;
        end
    end

    Sa = S(state,1);
    Sb = S(state,2); 
    Sc = S(state,3);

    x = x + (Sa-Sap)^2 + (Sb-Sbp)^2 + (Sc-Scp)^2 ;
    
    if ((state == 1 || state == 8) && (prev_state~=state))
        y = y + 1;
    end

    Sum = x ;
    Spikes = y;
end

== matlab function mpc_final/MATLAB Function1 ==
  data: Van input; Vs output; Vbn input; Vcn input
function Vs  = fcn(Van,Vbn,Vcn)

a=complex(cos(2*pi/3),sin(2*pi/3)); 
Vs =(2/3)*(Van+(a*Vbn)+((a^2)*Vcn)) ;
